simulink model "RobotX_DKin"  (R2024a)
settings: Solver=VariableStepAuto  StartTime=0.0  StopTime=inf  RelTol=1e-3  EnableMultiTasking=on
libraries: vrlib x8, simulink x7, aerolibconvert2 x6, RobotX_Lib x1
settings Model: Creator=jorgemartins  LastModifiedBy=margaridaestrela
settings SolverCC: AlgebraicLoopSolver=TrustRegion
settings DataIOCC: LimitDataPoints=on  ReturnWorkspaceOutputs=off
settings OptimizationCC: LifeSpan=inf
settings DebuggingCC: UnconnectedInputMsg=warning  UnconnectedOutputMsg=warning  UnconnectedLineMsg=warning  AllowSymbolicDim=off  SFUnexpectedBacktrackingDiag=warning  SFNoUnconditionalDefaultTransitionDiag=warning  SFExecutionAtInitializationDiag=none  ArithmeticOperatorsInVariantConditions=warning
settings ModelReferenceCC: EnableRefExpFcnMdlSchedulingChecks=on  PropagateSignalLabelsOutOfModel=off
settings SFSimCC: SimUseLocalCustomCode=off  CustomCodeUndefinedFunction=UseInterfaceOnly
settings RTWCC: RTWUseLocalCustomCode=off  GPUComputeCapability=3.5
settings CodeAppCC: StateflowObjectComments=on
settings GRTTargetCC: TargetLangStandard=C89/C90 (ANSI)
settings ConfigComp: CovMetricSettings=dw  CovSaveCumulativeToWorkspaceVar=on  CovSaveSingleToWorkspaceVar=on  CovExternalEMLEnable=off

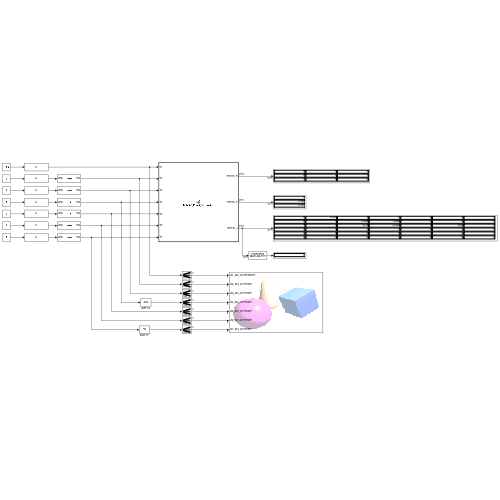
[thumbnail: Simulink's stored preview of the top-level diagram]
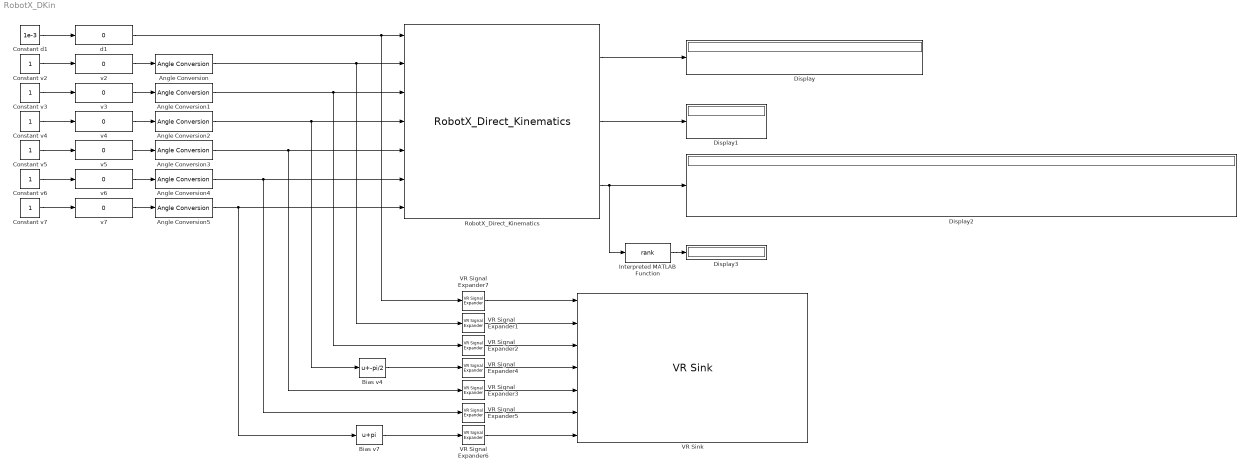
== system RobotX_DKin ==
  Angle Conversion{,1..5} (6 alike) : aerolibconvert2/Angle Conversion  IU=deg  OU=rad
  Bias v4 : Bias  Bias=-pi/2  SaturateOnIntegerOverflow=off
  Bias v7 : Bias  Bias=pi  SaturateOnIntegerOverflow=off
  Constant d1 : Constant  Value=1e-3
  Constant v{2..7} (6 alike) : Constant
  Display{,1..3} (4 alike) : Display
      Display settings: Format=decimal (Stored Integer)  Decimation=2
      Display1 settings: Format=decimal (Stored Integer)
      Display2 settings: Format=decimal (Stored Integer)
      Display3 settings: Format=decimal (Stored Integer)
  Interpreted MATLAB Function : MATLABFcn  MATLABFcn=rank
  RobotX_Direct_Kinematics : RobotX_Lib/RobotX_Direct_Kinematics  SystemSampleTime=-1  VariantActivationTime=update diagram  AllowFlexibleInterface=on  Latency=0  AutoFrameSizeCalculation=off
  VR Signal Expander{1..6} (6 alike) : vrlib/VR Signal Expander  outwidth=4  outidx=[4]
  VR Signal Expander7 : vrlib/VR Signal Expander  outwidth=3  outidx=[3]
  VR Sink : vrlib/VR Sink  InstantiateOnLoad=on  SampleTime=0.1  ViewEnable=on  RemoteChange=off  RemoteView=off  FieldsWritten=Jt1_DH_dv.translation.3.1.1.double#Jt2_DH_dv.rotation.4.1.1.double#Jt3_DH_dv.rotation.4.1.1.double#Jt4_DH_dv.rotation.4.1.1.double#Jt5_DH_dv.rotation.4.1.1.double#Jt6_DH_dv.rotation.4.1.1.double#Jt7_DH_dv.rotation.4.1.1.double  WorldFileName=vrrobot.wrl  WorldDescription=D-H Reference Frames for Virtual Reality Robot  AutoView=on  VideoDimensions=[]  AllowVariableSize=off
  d1 : simulink/Math Operations/Slider Gain  gain=0  low=-350  high=350
  v2 : simulink/Math Operations/Slider Gain  gain=0  low=-170  high=170
  v3 : simulink/Math Operations/Slider Gain  gain=0  low=-190  high=45
  v4 : simulink/Math Operations/Slider Gain  gain=0  low=-120  high=156
  v5 : simulink/Math Operations/Slider Gain  gain=0  low=-185  high=185
  v6 : simulink/Math Operations/Slider Gain  gain=0  low=-120  high=120
  v7 : simulink/Math Operations/Slider Gain  gain=0  low=-350  high=350
  wires:
  RobotX_Direct_Kinematics/1 -> Display/1
  RobotX_Direct_Kinematics/2 -> Display1/1
  Constant v3/1 -> v3/1
  Constant d1/1 -> d1/1
  d1/1 -> VR Signal Expander7/1, RobotX_Direct_Kinematics/1
  Constant v2/1 -> v2/1
  v2/1 -> Angle Conversion/1
  Constant v4/1 -> v4/1
  Constant v6/1 -> v6/1
  Constant v5/1 -> v5/1
  v5/1 -> Angle Conversion3/1
  v6/1 -> Angle Conversion4/1
  Constant v7/1 -> v7/1
  v7/1 -> Angle Conversion5/1
  RobotX_Direct_Kinematics/3 -> Interpreted MATLAB Function/1, Display2/1
  v3/1 -> Angle Conversion1/1
  v4/1 -> Angle Conversion2/1
  Bias v4/1 -> VR Signal Expander4/1
  Bias v7/1 -> VR Signal Expander6/1
  VR Signal Expander1/1 -> VR Sink/2
  VR Signal Expander2/1 -> VR Sink/3
  VR Signal Expander4/1 -> VR Sink/4
  VR Signal Expander3/1 -> VR Sink/5
  VR Signal Expander5/1 -> VR Sink/6
  VR Signal Expander6/1 -> VR Sink/7
  VR Signal Expander7/1 -> VR Sink/1
  Angle Conversion/1 -> VR Signal Expander1/1, RobotX_Direct_Kinematics/2
  Angle Conversion1/1 -> VR Signal Expander2/1, RobotX_Direct_Kinematics/3
  Angle Conversion2/1 -> Bias v4/1, RobotX_Direct_Kinematics/4
  Angle Conversion3/1 -> VR Signal Expander3/1, RobotX_Direct_Kinematics/5
  Angle Conversion4/1 -> VR Signal Expander5/1, RobotX_Direct_Kinematics/6
  Angle Conversion5/1 -> Bias v7/1, RobotX_Direct_Kinematics/7
  Interpreted MATLAB Function/1 -> Display3/1
